simulink model "Automatic_reclosing"  (R2023a)
settings: Solver=VariableStepAuto  StartTime=0.0  StopTime=1  MaxStep=1e-4  RelTol=1e-3
undefined symbols (not defined in the file): D1, Delta
libraries: spsThreePhaseSeriesRLCLoadLib x2, dspswit3 x1, spsDistributedParametersLineLib x1, spsThreePhaseTransformerTwoWindingsLib x1, spsThreePhaseVIMeasurementLib x1, spsThreePhaseBreakerLib x1, spsThreePhaseFaultLib x1, spsThreePhaseSourceLib x1, spspowerguiLib x1
settings Model: Creator=Lightrain  LastModifiedBy=Lightrain
settings DebuggingCC: IgnoredZcDiagnostic=none

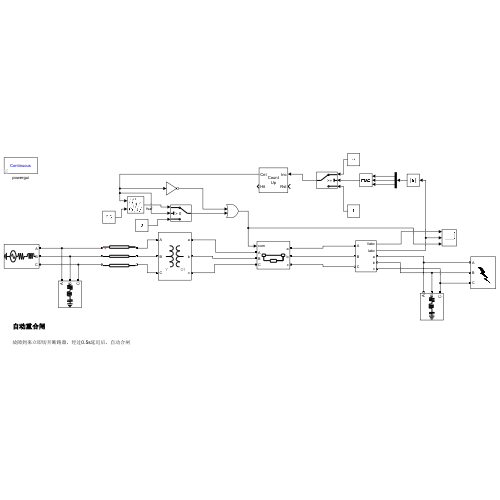
[thumbnail: Simulink's stored preview of the top-level diagram]
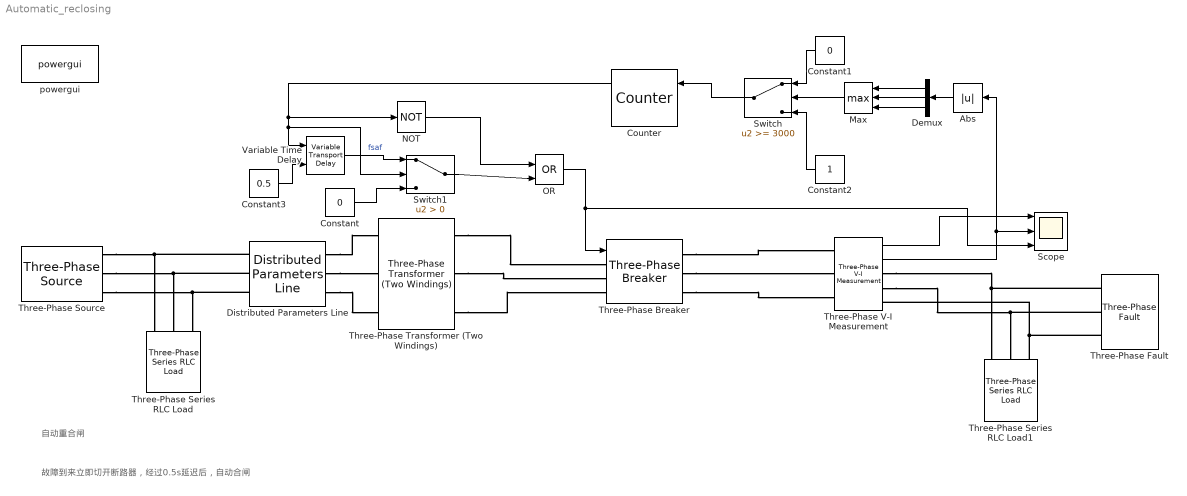
== system Automatic_reclosing ==
  note: 故障到来立即切开断路器，经过0.5s延迟后，自动合闸
  note: 自动重合闸
  Abs : Abs  SaturateOnIntegerOverflow=off
  Constant : Constant  Value=0
  Constant1 : Constant  Value=0
  Constant2 : Constant
  Constant3 : Constant  Value=0.5
  Counter : dspswit3/Counter  Direction=Up  CountEvent=Rising edge  CounterSize=User defined  MaxCount=255  InitialCount=0  Output=Count and Hit  HitValue=32  ResetInput=on  SamplesPerFrame=1  Ts=1  CntDtype=double  HitDtype=Logical
  Demux : Demux  Outputs=3
  Distributed Parameters Line : spsDistributedParametersLineLib/Distributed Parameters Line  Phases=3  Length=100  Frequency=60  Resistance=[0.01273 0.3864]  Inductance="[0.9337e-3  4.1264e-3]"  Capacitance=[12.74e-9 7.751e-9]  x1=[4.19993584791135e-10 488362.286919741 488362.28691975;314.159265358979 314.159265358979 314.159265358979;-1.99344511313911 0.361117350101404 -1.20967897669349]  x2=[7.38492134974472e-09 450824.244330738 450824.244330792;314.159265358979 314.159265358979 314.159265358979;-1.32183895688537 0.331542958547636 -1.23925336824719]  x3=[4.99891640153224e-11 1738.01563196616 1738.01563196596;314.159265358979 314.159265358979 314.159265358979;-2.57459442708176 1.09674118487029 -0.474055141925668]  x4=[4.81886994105295e-11 2579.88526313003 2579.88526312844;314.159265358979 314.159265358979 314.159265358979;0.373683824513142 -0.213875794173 -1.78467212096755]  x5=0.000565541566995742  V1=[4.2e-10 4.884e+05 4.884e+05;314.2 314.2 314.2;-1.993 0.3611 -1.21]  V2=[7.385e-09 4.508e+05 4.508e+05;314.2 314.2 314.2;-1.322 0.3315 -1.239]  I1=[4.999e-11 1738 1738;314.2 314.2 314.2;-2.575 1.097 -0.4741]  I2=[4.819e-11 2580 2580;314.2 314.2 314.2;0.3737 -0.2139 -1.785]  nHarmo=1  Measurements=None  Decoupling=off  VsMag0=0  VrMag0=0  VsAngle0=0  VrAngle0=0  IsMag0=0  IrMag0=0  IsAngle0=0  IrAngle0=0
      settings: LibrarySourceBlock=sps_lib/Power Grid Elements/Distributed Parameters Line
  Max : MinMax  Function=max  Inputs=3
  NOT : Logic  Operator=NOT  IconShape=distinctive  AllPortsSameDT=off  OutDataTypeStr=boolean
  OR : Logic  Operator=OR  IconShape=distinctive  AllPortsSameDT=off  OutDataTypeStr=boolean
  Scope : Scope  NumInputPorts=3
  Switch : Switch  Threshold=3000  SaturateOnIntegerOverflow=off  InputSameDT=off
  Switch1 : Switch  Criteria=u2 > Threshold  SaturateOnIntegerOverflow=off  InputSameDT=off
  Three-Phase Series RLC Load : spsThreePhaseSeriesRLCLoadLib/Three-Phase Series RLC Load  LConnTagsString=A|B|C  Configuration=Y (grounded)  NominalVoltage=1000  Vabc=[1e3 1e3 1e3]  Vabcp=[1e3 1e3 1e3]  NominalFrequency=50  UnbalancedPower=off  ActivePower=10e3  InductivePower=100  CapacitivePower=100  Pabc=[10e3 9e3 11e3]  QLabc=[100 90 110]  QCabc=[100 90 110]  Pabcp=[10e3 9e3 11e3]  QLabcp=[100 90 110]  QCabcp=[100 90 110]  Measurements=None  LoadType=constant Z
  Three-Phase Series RLC Load1 : spsThreePhaseSeriesRLCLoadLib/Three-Phase Series RLC Load  LConnTagsString=A|B|C  Configuration=Y (grounded)  NominalVoltage=1000  Vabc=[1e3 1e3 1e3]  Vabcp=[1e3 1e3 1e3]  NominalFrequency=50  UnbalancedPower=off  ActivePower=50e3  InductivePower=100  CapacitivePower=100  Pabc=[10e3 9e3 11e3]  QLabc=[100 90 110]  QCabc=[100 90 110]  Pabcp=[10e3 9e3 11e3]  QLabcp=[100 90 110]  QCabcp=[100 90 110]  Measurements=None  LoadType=constant Z
  Three-Phase Transformer (Two Windings) : spsThreePhaseTransformerTwoWindingsLib/Three-Phase Transformer (Two Windings)  Winding1Connection=Y  Winding2Connection=Delta (D1)  CoreType=Three single-phase transformers  SetSaturation=off  Hysteresis=off  DataFile='hysteresis'  SetInitialFlux=off  Measurements=None  UNITS=pu  NominalPower=[ 250e6 , 60 ]  Winding1=[ 735e3 , 0.002 , 0.08 ]  Winding2=[ 315e3 , 0.002 , 0.08 ]  Rm=500  Lm=500  L0=0.5  Saturation=[ 0,0 ; 0.0024,1.2 ; 1.0,1.52 ]  InitialFluxes=[ 0.8 , -0.8 , 0.7 ]  BreakLoop=off  DiscreteSolver=Trapezoidal iterative  DataType=off  TransfoNumber=1
  Three-Phase V-I Measurement : spsThreePhaseVIMeasurementLib/Three-Phase V-I Measurement  VoltageMeasurement=phase-to-phase  SetLabelV=off  LabelV=Vabc  Vpu=off  VpuLL=off  CurrentMeasurement=yes  SetLabelI=off  LabelI=Iabc  Ipu=off  Pbase=100e6  Vbase=500e3  OutputType=Complex  PhasorSimulation=off  PSBequivalent=0
  Three-Phase Breaker : spsThreePhaseBreakerLib/Three-Phase Breaker  InitialState=closed  SwitchA=on  SwitchB=on  SwitchC=on  SwitchTimes="[1/60  5/60]"  External=on  BreakerResistance=0.01  SnubberResistance=1e6  SnubberCapacitance=inf  Measurements=None
  Three-Phase Fault : spsThreePhaseFaultLib/Three-Phase Fault  InitialStates=0  FaultA=on  FaultB=on  FaultC=on  GroundFault=off  SwitchTimes=[0.2 0.3]  External=off  SwitchStatus=NaN  FaultResistance=0.001  GroundResistance=0.01  SnubberResistance=1e6  SnubberCapacitance=inf  Measurements=None
  Three-Phase Source : spsThreePhaseSourceLib/Three-Phase Source  InternalConnection=Yg  VoltagePhases=off  Voltage=500e3  PhaseAngle=0  Voltage_phases=[25e3 25e3 25e3]/sqrt(3)  PhaseAngles_phases=[0 -120 +120]  Frequency=50  NonIdealSource=on  SpecifyImpedance=off  Resistance=0.8929  Inductance=16.58e-3  ShortCircuitLevel=100e6  BaseVoltage=25e3  XRratio=7  BusType=swing  Pref=10e3  Qref=0  Prefabc=[10e3, 10e3, 10e3]  Qrefabc=[0, 0, 0]  Qmin=-inf  Qmax=inf
  Variable Time Delay : VariableTransportDelay  MaximumDelay=10
  powergui : spspowerguiLib/powergui  Priority=1  SimulationMode=Continuous  SampleTime=50e-6  frequency=60  Iterations=50  frequencyindice=60  Pbase=100e6  ErrMax=1e-4  UnitsV=kV  UnitsW=MW  buscounter=0  FunctionMessages=off  echomessages=off  EnableUseOfTLC=off  CurrentSourceSwitches=off  DisableSnubberDevices=off  DisableRonSwitches=off  DisableVfSwitches=off  DisplayEquations=off  AutomaticDiscreteSolvers=off  SolverType=Tustin/Backward Euler (TBE)  Interpol=off  ExternalGateDelay=off  methode=off  Ts=100  x0status=blocks  SPID=on  SwTol=0  HookPort=off  NonlinearTolerance=1e-4  nMaxIteration=100  ContinueOnMaxIteration=off  RestoreLinks=warning  ResistiveCurrentMeasurement=off  Frange=[0:2:500]  Ylog=off  Xlog=on  ShowGrid=off  save=off  variable=ZData  structure=0  ZoomFFT=off  StartTime=0.0  cycles=1  DisplayStyle=1  fundamental=60  FreqAxis=off  MaxFrequency=1000  frequencyindicesteady=1  RmsSteady=1  display=off
  wires:
  Three-Phase V-I Measurement/1 -> Scope/1
  Three-Phase V-I Measurement/2 -> Abs/1, Scope/2
  Abs/1 -> Demux/1
  Demux/1 -> Max/1
  Demux/2 -> Max/2
  Demux/3 -> Max/3
  Max/1 -> Switch/2
  Constant1/1 -> Switch/1
  Constant2/1 -> Switch/3
  Switch/1 -> Counter/1
  Counter/1 -> Switch1/2, Variable Time Delay/1, NOT/1
  Constant3/1 -> Variable Time Delay/2
  NOT/1 -> OR/1
  OR/1 -> Scope/3, Three-Phase Breaker/1
  Constant/1 -> Switch1/3
  Switch1/1 -> OR/2
  Variable Time Delay/1 -> Switch1/1  "fsaf"
  connections:
  Three-Phase Source/RConn1 -- Distributed Parameters Line/LConn1 -- Three-Phase Series RLC Load/LConn1
  Three-Phase Source/RConn2 -- Distributed Parameters Line/LConn2 -- Three-Phase Series RLC Load/LConn2
  Three-Phase Source/RConn3 -- Distributed Parameters Line/LConn3 -- Three-Phase Series RLC Load/LConn3
  Three-Phase Breaker/RConn2 -- Three-Phase V-I Measurement/LConn2
  Three-Phase Breaker/RConn1 -- Three-Phase V-I Measurement/LConn1
  Three-Phase Breaker/RConn3 -- Three-Phase V-I Measurement/LConn3
  Three-Phase V-I Measurement/RConn1 -- Three-Phase Fault/LConn1 -- Three-Phase Series RLC Load1/LConn1
  Three-Phase V-I Measurement/RConn2 -- Three-Phase Fault/LConn2 -- Three-Phase Series RLC Load1/LConn2
  Three-Phase Series RLC Load1/LConn3 -- Three-Phase Fault/LConn3 -- Three-Phase V-I Measurement/RConn3
  Distributed Parameters Line/RConn2 -- Three-Phase Transformer (Two Windings)/LConn2
  Distributed Parameters Line/RConn3 -- Three-Phase Transformer (Two Windings)/LConn3
  Distributed Parameters Line/RConn1 -- Three-Phase Transformer (Two Windings)/LConn1
  Three-Phase Transformer (Two Windings)/RConn2 -- Three-Phase Breaker/LConn2
  Three-Phase Transformer (Two Windings)/RConn3 -- Three-Phase Breaker/LConn3
  Three-Phase Transformer (Two Windings)/RConn1 -- Three-Phase Breaker/LConn1
